simulink model "joint_space_inv_dyn"  (R2021b)
settings: Solver=FixedStepAuto  StartTime=0.0  StopTime=5  FixedStep=Ts  RelTol=1e-3
undefined symbols (not defined in the file): dqi, KD, KP, myRobot, qi, wrongModel
libraries: vrlib x1
settings Model: Creator=simon  LastModifiedBy=luigi
settings SolverCC: ZeroCrossControl=DisableAll  AlgebraicLoopSolver=TrustRegion
settings DebuggingCC: SFMachineParentedDataDiag=warning

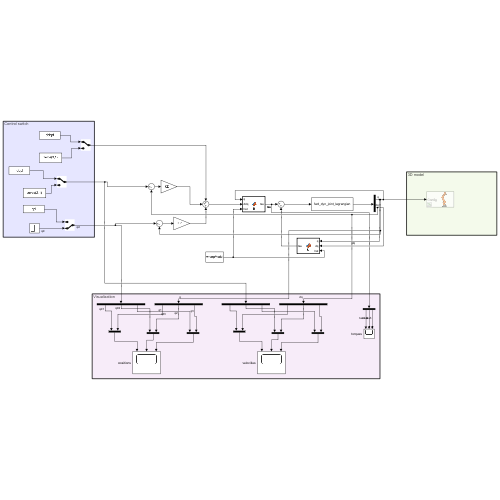
[thumbnail: Simulink's stored preview of the top-level diagram]
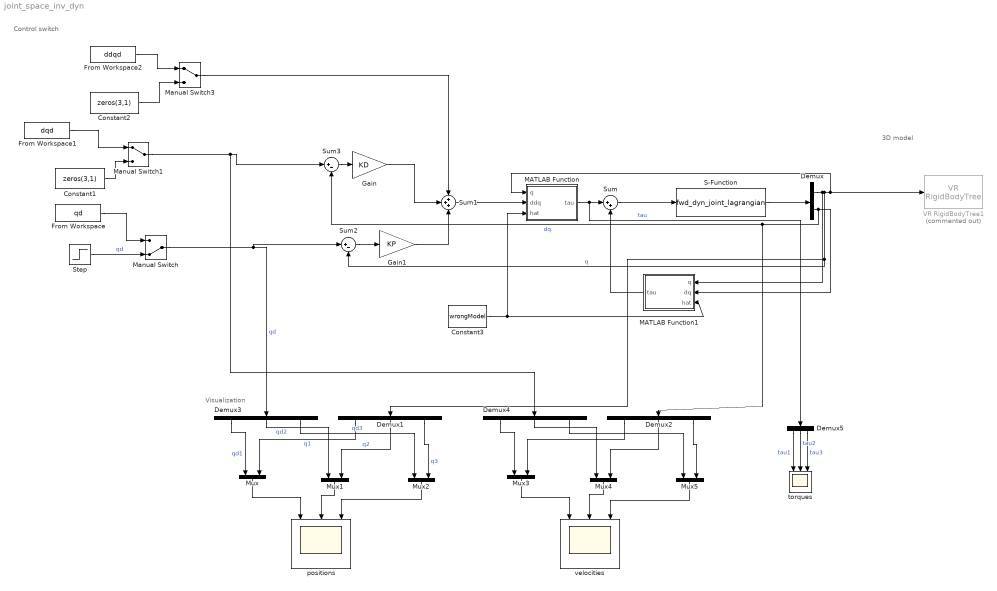
== system joint_space_inv_dyn ==
  note: 3D model
  note: Visualization
  note: Control switch
  Constant1 : Constant  Value=zeros(3,1)
  Constant2 : Constant  Value=zeros(3,1)
  Constant3 : Constant  Value=wrongModel
  Demux : Demux  Outputs=2
  Demux{1..4} (4 alike) : Demux  Outputs=myRobot.N
  Demux5 : Demux  Outputs=3
  From Workspace : FromWorkspace  VariableName=qd
  From Workspace1 : FromWorkspace  VariableName=dqd
  From Workspace2 : FromWorkspace  VariableName=ddqd
  Gain : Gain  Gain=KD
  Gain1 : Gain  Gain=KP
  MATLAB Function : MATLAB Function  TreatAsAtomicUnit=on
  MATLAB Function1 : MATLAB Function  TreatAsAtomicUnit=on
  Manual Switch : ManualSwitch  CurrentSetting=0
  Manual Switch1 : ManualSwitch
  Manual Switch3 : ManualSwitch
  Mux{,1..5} (6 alike) : Mux  Inputs=2
  S-Function : S-Function  FunctionName=fwd_dyn_joint_lagrangian  Parameters=myRobot,qi,dqi  SFunctionDeploymentMode=off  EnableBusSupport=off
  Step : Step  Time=0  After=ones(3,1)  SampleTime=0
  Sum : Sum  Inputs=|++
  Sum1 : Sum  Inputs=+++
  Sum2 : Sum  Inputs=|+-
  Sum3 : Sum  Inputs=|+-
  VR RigidBodyTree1 : vrlib/VR RigidBodyTree  Commented=on  RBT=rbt  useRBT=on  Ts=-1  ForceViewerOpen=on
      settings: SourceProductBaseCode=SL
  positions : Scope  NumInputPorts=3
  torques : Scope  NumInputPorts=3
  velocities : Scope  NumInputPorts=3
  wires:
  Demux/1 -> Demux1/1, Sum2/2, VR RigidBodyTree1/1, MATLAB Function/1(q), MATLAB Function1/1(q)  "q"
  Sum2/1 -> Gain1/1
  Gain1/1 -> Sum1/3
  Demux/2 -> Demux2/1, Sum3/2, MATLAB Function1/2(dq)  "dq"
  Constant3/1 -> MATLAB Function/3(hat), MATLAB Function1/3(hat)
  Sum1/1 -> MATLAB Function/2(ddq)
  Sum3/1 -> Gain/1
  MATLAB Function1/1(tau) -> Sum/2
  Gain/1 -> Sum1/2
  MATLAB Function/1(tau) -> Demux5/1, Sum/1  "tau"
  S-Function/1 -> Demux/1
  Sum/1 -> S-Function/1
  Manual Switch3/1 -> Sum1/1
  Manual Switch/1 -> Demux3/1, Sum2/1  "qd"
  Constant2/1 -> Manual Switch3/2
  From Workspace/1 -> Manual Switch/1
  Constant1/1 -> Manual Switch1/2
  Step/1 -> Manual Switch/2  "qd"
  From Workspace1/1 -> Manual Switch1/1
  From Workspace2/1 -> Manual Switch3/1
  Manual Switch1/1 -> Demux4/1, Sum3/1
  Demux4/3 -> Mux5/1
  Demux2/2 -> Mux4/2
  Demux4/2 -> Mux4/1
  Mux/1 -> positions/1
  Demux1/1 -> Mux/2  "q1"
  Demux3/3 -> Mux2/1  "qd3"
  Demux4/1 -> Mux3/1
  Mux5/1 -> velocities/3
  Demux1/3 -> Mux2/2  "q3"
  Demux5/1 -> torques/1  "tau1"
  Demux2/3 -> Mux5/2
  Mux1/1 -> positions/2
  Mux2/1 -> positions/3
  Mux3/1 -> velocities/1
  Demux2/1 -> Mux3/2
  Demux5/3 -> torques/3  "tau3"
  Demux5/2 -> torques/2  "tau2"
  Demux3/1 -> Mux/1  "qd1"
  Demux3/2 -> Mux1/1  "qd2"
  Demux1/2 -> Mux1/2  "q2"
  Mux4/1 -> velocities/2

== matlab function joint_space_inv_dyn/MATLAB Function ==
  data: q input size=3; tau output; ddq input size=3; hat input
function tau = B(q, ddq, hat)
if hat == 0
    B = getB(q);
else
    B = getBHat(q);
end

tau = B*ddq;

== matlab function joint_space_inv_dyn/MATLAB Function1 ==
  data: q input size=3; tau output; dq input size=3; hat input
function tau = N(q, dq, hat)
if hat == 0
    tau = getN(q, dq);
else
    tau = getNHat(q, dq);
end
